simulink model "enabledSubsystem_example2"  (R2017a)
settings: Solver=VariableStepAuto  StartTime=0.0  StopTime=20  RelTol=1e-3
settings Model: Creator=edward  LastModifiedBy=edward

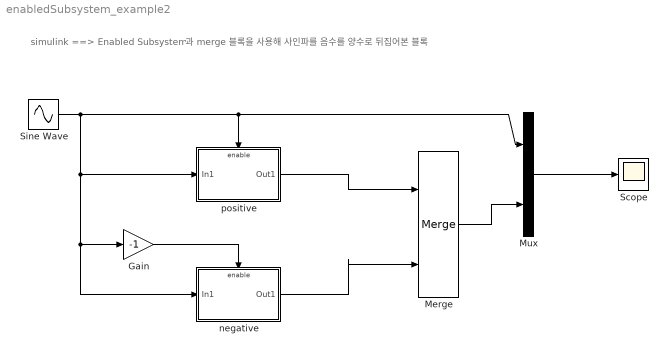
== system enabledSubsystem_example2 ==
  note: simulink ==> Enabled Subsystem과 merge 블록을 사용해 사인파를 음수를 양수로 뒤집어본 블록
  Gain : Gain  Gain=-1
  Merge : Merge
  Mux : Mux  Inputs=2
  Scope : Scope
  Sine Wave : Sin  SampleTime=0
  "negative " : Subsystem
  "positive " : Subsystem
  wires:
  Sine Wave/1 -> "positive "/1(In1), "negative "/1(In1), Gain/1, Mux/1, "positive "/Enable
  "positive "/1(Out1) -> Merge/1
  Gain/1 -> "negative "/Enable
  "negative "/1(Out1) -> Merge/2
  Merge/1 -> Mux/2
  Mux/1 -> Scope/1

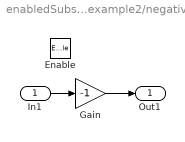
== system enabledSubsystem_example2/negative  ==
  In1 : Inport
  Enable : EnablePort
  Gain : Gain  Gain=-1
  Out1 : Outport
  wires:
  In1/1 -> Gain/1
  Gain/1 -> Out1/1

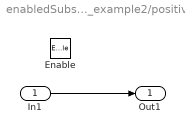
== system enabledSubsystem_example2/positive  ==
  In1 : Inport
  Enable : EnablePort
  Out1 : Outport
  wires:
  In1/1 -> Out1/1
